simulink model "ACS"  (R2023b)
settings: Solver=FixedStepDiscrete  StartTime=0.0  StopTime=10000  FixedStep=0.01  MaxStep=10  RelTol=1e-5  AbsTol=1e-5  EnableMultiTasking=on
InitFcn:
  | initialization
undefined symbols (not defined in the file): A, AE, air_density, altitude, c_diffus, c_spec, CD, Cell_Area, CM_mm01, CM_mm02, CM_mm03, CO_mm01, CO_mm02, CO_mm03, cos50, cosines, dip_coel, dip_long, DiscIntNeverNeededParam, E_EOL, H0, inc, Inertia_tensor, K_l, k_pb, k_pe, kelly, light_speed, m_m, M_SR, magnitude, MM_Working, MT_Working, N_B, Ncell_Xn, Ncell_Xp, Ncell_Yn, Ncell_Yp, Ncell_Zn, Ncell_Zp, NX, NY, NZ, omega_BI_B0, omega_e, omega_o, omega_tx, omega_ty, omega_tz, quat_0, r, r_cm_B, r_cp_a_B, r_cp_s_B, RAAN_rt, Re, t0, TA_0, theta_g0
libraries: simulink x20, vrlib x5
(part 2 of 3)

== system ACS/Satellite/Magnetorquers/Magnetorquers4 ==
  MT : Inport
  Abs1 : Abs  SaturateOnIntegerOverflow=off
  Constant1 : Constant  Value=0
  Constant4 : Constant  Value=0.0511597
  Constant5 : Constant  Value=24.7613/15/22
  Discrete-Time Integrator1 : DiscreteIntegrator  InitialConditionSource=external  SampleTime=-1  ICPrevOutput=DiscIntNeverNeededParam  ICPrevScaledInput=DiscIntNeverNeededParam
  Gain5 : Gain  Gain=1/15
  Gain6 : Gain  Gain=0.06
  Gain7 : Gain  Gain=22
  Product : Product  Inputs=*/
  Product1 : Product  Inputs=*/
  Sum : Sum  Inputs=+-
  MM_Am2 : Outport  VectorParamsAs1DForOutWhenUnconnected=off
  MM_W : Outport  Port=2  VectorParamsAs1DForOutWhenUnconnected=off
  wires:
  MT/1 -> Product/1
  Constant4/1 -> Product1/2
  Constant1/1 -> Discrete-Time Integrator1/2
  Discrete-Time Integrator1/1 -> MM_Am2/1, Abs1/1, Product1/1
  Product/1 -> Sum/1
  Sum/1 -> Discrete-Time Integrator1/1
  Product1/1 -> Sum/2
  Constant5/1 -> Product/2
  Abs1/1 -> Gain5/1
  Gain5/1 -> Gain6/1
  Gain6/1 -> Gain7/1
  Gain7/1 -> MM_W/1

== system ACS/Satellite/OBC/Data Adquisition ==
  PP_W : Inport
  PD_V : Inport  Port=2
  B_b_V : Inport  Port=3
  Bus Creator : BusCreator  Inputs=3
  Bus Selector : BusSelector  OutputSignals=B_MM1,B_MM2,B_MM3
  Constant : Constant  Value=-960.9  OutDataTypeStr=single
  Constant1 : Constant  Value=-960.9  OutDataTypeStr=single
  Constant2 : Constant  Value=1975.166667  OutDataTypeStr=single
  Gain1 : Gain  Gain=363.6733333
  Gain3 : Gain  Gain=1147.5
  Gain4 : Gain  Gain=1147.5
  Saturation : Saturate  UpperLimit=4.4  LowerLimit=1  ZeroCross=off
  Saturation1 : Saturate  UpperLimit=4.4  LowerLimit=1  ZeroCross=off
  Saturation2 : Saturate  UpperLimit=5.6  LowerLimit=-5.4  ZeroCross=off
  Sum : Sum
  Sum1 : Sum
  Sum2 : Sum
  PP_UPC : Outport  VectorParamsAs1DForOutWhenUnconnected=off
  PD_UPC : Outport  Port=2  VectorParamsAs1DForOutWhenUnconnected=off
  B_b_UPC : Outport  Port=3  VectorParamsAs1DForOutWhenUnconnected=off
  wires:
  B_b_V/1 -> Bus Selector/1
  Bus Creator/1 -> B_b_UPC/1
  PD_V/1 -> PD_UPC/1
  PP_W/1 -> PP_UPC/1
  Bus Selector/1 -> Saturation/1  "<B_MM1>"
  Bus Selector/2 -> Saturation1/1  "<B_MM2>"
  Bus Selector/3 -> Saturation2/1  "<B_MM3>"
  Saturation/1 -> Gain3/1
  Sum/1 -> Bus Creator/1
  Saturation1/1 -> Gain4/1
  Saturation2/1 -> Gain1/1
  Sum2/1 -> Bus Creator/3
  Sum1/1 -> Bus Creator/2
  Gain3/1 -> Sum/1
  Gain4/1 -> Sum1/1
  Gain1/1 -> Sum2/1
  Constant/1 -> Sum/2
  Constant1/1 -> Sum1/2
  Constant2/1 -> Sum2/2

== system ACS/Satellite/OBC/Experimentall Attitude Control ==
  PP_UPC : Inport
  PD_UPC : Inport  Port=2
  B_b_UPC : Inport  Port=3
  Constant1 : Constant  Value=0  OutDataTypeStr=single
  Constant3 : Constant  Value=0  OutDataTypeStr=single
  Terminator1 : Terminator
  Terminator2 : Terminator
  Terminator3 : Terminator
  MT : Outport  VectorParamsAs1DForOutWhenUnconnected=off
  RW : Outport  Port=2  VectorParamsAs1DForOutWhenUnconnected=off
  wires:
  B_b_UPC/1 -> Terminator3/1
  PD_UPC/1 -> Terminator1/1
  PP_UPC/1 -> Terminator2/1
  Constant3/1 -> MT/1
  Constant1/1 -> RW/1

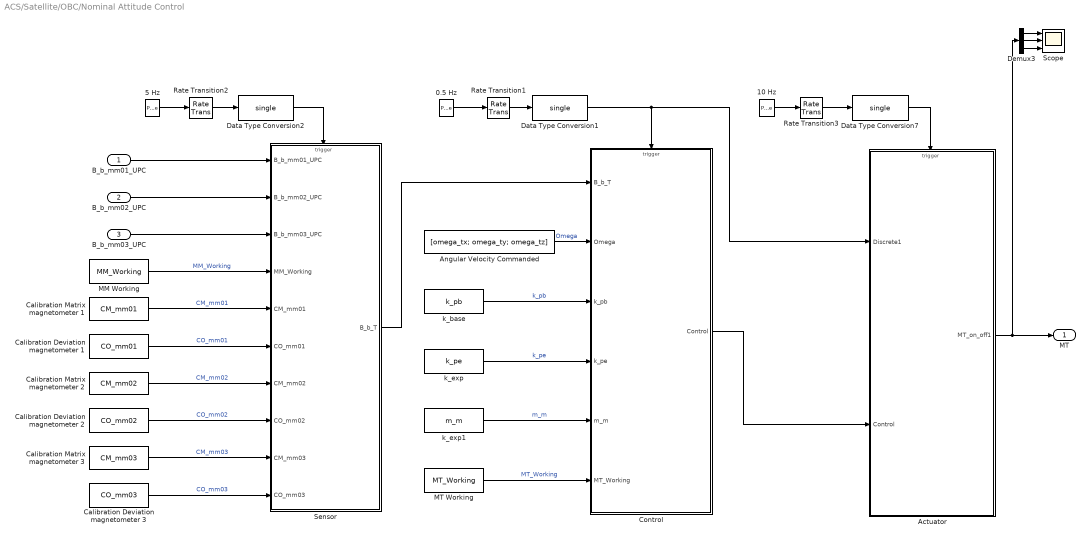
== system ACS/Satellite/OBC/Nominal Attitude Control ==
  B_b_mm01_UPC : Inport
  B_b_mm02_UPC : Inport  Port=2
  B_b_mm03_UPC : Inport  Port=3
  " 5 Hz" : DiscretePulseGenerator  PulseType=Time based  Period=0.2  PulseWidth=50
  0.5 Hz : DiscretePulseGenerator  PulseType=Time based  PulseWidth=25  PhaseDelay=1
  10 Hz : DiscretePulseGenerator  PulseType=Time based  Period=0.2  PulseWidth=50
  Actuator : Subsystem
  Angular Velocity Commanded : Constant  Value=[omega_tx; omega_ty; omega_tz]  OutDataTypeStr=single
  Calibration Deviation magnetometer 1 : Constant  Value=CO_mm01  OutDataTypeStr=single
  Calibration Deviation magnetometer 2 : Constant  Value=CO_mm02  OutDataTypeStr=single
  Calibration Deviation magnetometer 3 : Constant  Value=CO_mm03  OutDataTypeStr=single
  Calibration Matrix magnetometer 1 : Constant  Value=CM_mm01  OutDataTypeStr=single
  Calibration Matrix magnetometer 2 : Constant  Value=CM_mm02  OutDataTypeStr=single
  Calibration Matrix magnetometer 3 : Constant  Value=CM_mm03  OutDataTypeStr=single
  Control : Subsystem
  Data Type Conversion1 : DataTypeConversion  OutDataTypeStr=single  SampleTime=0.1  SaturateOnIntegerOverflow=off  RndMeth=Floor
  Data Type Conversion2 : DataTypeConversion  OutDataTypeStr=single  SampleTime=0.1  SaturateOnIntegerOverflow=off  RndMeth=Floor
  Data Type Conversion7 : DataTypeConversion  OutDataTypeStr=single  SampleTime=0.1  SaturateOnIntegerOverflow=off  RndMeth=Floor
  Demux3 : Demux  Outputs=3
  MM Working : Constant  Value=MM_Working  OutDataTypeStr=single
  MT Working : Constant  Value=MT_Working  OutDataTypeStr=single
  Rate Transition1 : RateTransition  OutPortSampleTime=0.1
  Rate Transition2 : RateTransition  OutPortSampleTime=0.1
  Rate Transition3 : RateTransition  OutPortSampleTime=0.1
  Scope : Scope  NumInputPorts=3
  Sensor : Subsystem
  k_base : Constant  Value=k_pb  OutDataTypeStr=single
  k_exp : Constant  Value=k_pe  OutDataTypeStr=single
  k_exp1 : Constant  Value=m_m  OutDataTypeStr=single
  MT : Outport  VectorParamsAs1DForOutWhenUnconnected=off
  wires:
  Control/1(Control) -> Actuator/2(Control)
  0.5 Hz/1 -> Rate Transition1/1
  10 Hz/1 -> Rate Transition3/1
  Sensor/1(B_b_T) -> Control/1(B_b_T)
  B_b_mm01_UPC/1 -> Sensor/1(B_b_mm01_UPC)
  Data Type Conversion7/1 -> Actuator/Trigger
  Data Type Conversion1/1 -> Control/Trigger, Actuator/1(Discrete1)
  " 5 Hz"/1 -> Rate Transition2/1
  Data Type Conversion2/1 -> Sensor/Trigger
  MM Working/1 -> Sensor/4(MM_Working)  "MM_Working"
  Calibration Matrix magnetometer 1/1 -> Sensor/5(CM_mm01)  "CM_mm01"
  Calibration Deviation magnetometer 1/1 -> Sensor/6(CO_mm01)  "CO_mm01"
  Calibration Matrix magnetometer 2/1 -> Sensor/7(CM_mm02)  "CM_mm02"
  Calibration Deviation magnetometer 2/1 -> Sensor/8(CO_mm02)  "CO_mm02"
  Calibration Matrix magnetometer 3/1 -> Sensor/9(CM_mm03)  "CM_mm03"
  Calibration Deviation magnetometer 3/1 -> Sensor/10(CO_mm03)  "CO_mm03"
  Angular Velocity Commanded/1 -> Control/2(Omega)  "Omega"
  k_base/1 -> Control/3(k_pb)  "k_pb"
  k_exp/1 -> Control/4(k_pe)  "k_pe"
  k_exp1/1 -> Control/5(m_m)  "m_m"
  MT Working/1 -> Control/6(MT_Working)  "MT_Working"
  B_b_mm02_UPC/1 -> Sensor/2(B_b_mm02_UPC)
  B_b_mm03_UPC/1 -> Sensor/3(B_b_mm03_UPC)
  Rate Transition2/1 -> Data Type Conversion2/1
  Rate Transition1/1 -> Data Type Conversion1/1
  Rate Transition3/1 -> Data Type Conversion7/1
  Actuator/1(MT_on_off1) -> MT/1, Demux3/1
  Demux3/3 -> Scope/3
  Demux3/2 -> Scope/2
  Demux3/1 -> Scope/1

== system ACS/Satellite/Photodiodes/Measurements ==
  V : Inport
  Trigger : TriggerPort  VariantControl=(inherit)
  V_V : Outport  VectorParamsAs1DForOutWhenUnconnected=off
  wires:
  V/1 -> V_V/1

== system ACS/Satellite/Photodiodes/Sun ==
  Sol_b_W : Inport
  Add : Sum  Inputs=+++
  Add1 : Sum  Inputs=2
  Compare To Zero : simulink/Logic and Bit Operations/Compare To Zero  relop===  OutDataTypeStr=uint8  ZeroCross=off
  Demux : Demux  Outputs=3
  Math Function : Math  Operator=magnitude^2  SignedPower=on
  Math Function1 : Math  Operator=magnitude^2  SignedPower=on
  Math Function2 : Math  Operator=magnitude^2  SignedPower=on
  Math Function3 : Math  Operator=sqrt  SignedPower=on
  Product4 : Product  Inputs=*/  RndMeth=Zero
  Solar_Direction_b : Outport  VectorParamsAs1DForOutWhenUnconnected=off
  Solar_Flux_W : Outport  Port=2  VectorParamsAs1DForOutWhenUnconnected=off
  wires:
  Demux/1 -> Math Function/1
  Demux/2 -> Math Function1/1
  Math Function/1 -> Add/1
  Math Function1/1 -> Add/2
  Add/1 -> Math Function3/1
  Math Function3/1 -> Add1/1, Solar_Flux_W/1, Compare To Zero/1
  Demux/3 -> Math Function2/1
  Math Function2/1 -> Add/3
  Sol_b_W/1 -> Product4/1, Demux/1
  Product4/1 -> Solar_Direction_b/1
  Add1/1 -> Product4/2
  Compare To Zero/1 -> Add1/2

== system ACS/Satellite/Photodiodes/Voltage ==
  note: fi: angle between earth-sun vector and
      | normal vector of the solar array
  Earth-Sun B : Inport
  Solar Constant : Inport  Port=2
  eclipse : Inport  Port=3
  Constant1 : Constant  Value=NZ
  Constant2 : Constant  Value=NY
  Constant3 : Constant  Value=NX
  Dot Product1 : DotProduct  OutDataTypeStr=Inherit: Inherit via internal rule
  Dot Product2 : DotProduct  OutDataTypeStr=Inherit: Inherit via internal rule
  Dot Product3 : DotProduct  OutDataTypeStr=Inherit: Inherit via internal rule
  Power Generated : Subsystem
  Product3 : Product  Inputs=**  RndMeth=Zero
  factor of view X : Subsystem
  factor of view Y : Subsystem
  factor of view Z : Subsystem
  norm : Subsystem
  norm1 : Subsystem
  norm2 : Subsystem
  norm3 : Subsystem
  norm4 : Subsystem
  norm5 : Subsystem
  PD_V : Outport  VectorParamsAs1DForOutWhenUnconnected=off
  wires:
  norm3/1(2) -> Dot Product2/2
  norm2/1(2) -> Dot Product2/1
  norm1/1(2) -> Dot Product1/2
  norm/1(2) -> Dot Product1/1
  factor of view Z/1(FV) -> Power Generated/3(Cos fi NZ)
  factor of view Y/1(FV) -> Power Generated/2(Cos fi NY)
  Dot Product2/1 -> factor of view Z/1(cos (fi))  "cos fi"
  Dot Product1/1 -> factor of view Y/1(cos (fi))  "cos fi"
  Constant1/1 -> norm2/1(1)
  Constant2/1 -> norm/1(1)
  norm5/1(2) -> Dot Product3/2
  norm4/1(2) -> Dot Product3/1
  Dot Product3/1 -> factor of view X/1(cos (fi))  "cos fi"
  Constant3/1 -> norm4/1(1)
  Earth-Sun B/1 -> norm5/1(1), norm1/1(1), norm3/1(1)
  factor of view X/1(FV) -> Power Generated/1(Cos fi NX)
  Power Generated/1(Voltage) -> Product3/1
  Solar Constant/1 -> Power Generated/4(Solar_constant)
  Product3/1 -> PD_V/1
  eclipse/1 -> Product3/2

== system ACS/Satellite/Solar_Panels/Measurements ==
  V : Inport
  Trigger : TriggerPort  TriggerType=falling  VariantControl=(inherit)
  V_V : Outport  VectorParamsAs1DForOutWhenUnconnected=off
  wires:
  V/1 -> V_V/1

== system ACS/Satellite/Solar_Panels/Power ==
  note: fi: angle between earth-sun vector and
      | normal vector of the solar array
  Earth-Sun B : Inport
  Solar Constant : Inport  Port=2
  eclipse : Inport  Port=3
  Constant1 : Constant  Value=NZ
  Constant2 : Constant  Value=NY
  Constant3 : Constant  Value=NX
  Dot Product1 : DotProduct  OutDataTypeStr=Inherit: Inherit via internal rule
  Dot Product2 : DotProduct  OutDataTypeStr=Inherit: Inherit via internal rule
  Dot Product3 : DotProduct  OutDataTypeStr=Inherit: Inherit via internal rule
  Power Generated : Subsystem
  Product2 : Product  Inputs=**  RndMeth=Zero
  factor of view X : Subsystem
  factor of view Y : Subsystem
  factor of view Z : Subsystem
  norm : Subsystem
  norm1 : Subsystem
  norm2 : Subsystem
  norm3 : Subsystem
  norm4 : Subsystem
  norm5 : Subsystem
  Power_each_W : Outport  VectorParamsAs1DForOutWhenUnconnected=off
  wires:
  factor of view X/1(FV) -> Power Generated/1(Cos fi NX)
  Earth-Sun B/1 -> norm3/1(1), norm1/1(1), norm5/1(1)
  Constant3/1 -> norm4/1(1)
  Dot Product3/1 -> factor of view X/1(cos (fi))  "cos fi"
  norm4/1(2) -> Dot Product3/1
  norm5/1(2) -> Dot Product3/2
  Constant2/1 -> norm/1(1)
  Constant1/1 -> norm2/1(1)
  Dot Product1/1 -> factor of view Y/1(cos (fi))  "cos fi"
  Dot Product2/1 -> factor of view Z/1(cos (fi))  "cos fi"
  factor of view Y/1(FV) -> Power Generated/2(Cos fi NY)
  factor of view Z/1(FV) -> Power Generated/3(Cos fi NZ)
  norm/1(2) -> Dot Product1/1
  norm1/1(2) -> Dot Product1/2
  norm2/1(2) -> Dot Product2/1
  norm3/1(2) -> Dot Product2/2
  Solar Constant/1 -> Power Generated/4(Solar Constant)
  eclipse/1 -> Product2/2
  Product2/1 -> Power_each_W/1
  Power Generated/1(Power_each_W) -> Product2/1

== system ACS/Satellite/Solar_Panels/Power Generated ==
  Sol_b_W : Inport
  Add : Sum  Inputs=+++
  Add1 : Sum  Inputs=2
  Compare To Zero : simulink/Logic and Bit Operations/Compare To Zero  relop===  OutDataTypeStr=uint8  ZeroCross=off
  Demux : Demux  Outputs=3
  Math Function : Math  Operator=magnitude^2  SignedPower=on
  Math Function1 : Math  Operator=magnitude^2  SignedPower=on
  Math Function2 : Math  Operator=magnitude^2  SignedPower=on
  Math Function3 : Math  Operator=sqrt  SignedPower=on
  Product4 : Product  Inputs=*/  RndMeth=Zero
  Solar_Direction_b : Outport  VectorParamsAs1DForOutWhenUnconnected=off
  Solar_Flux_W : Outport  Port=2  VectorParamsAs1DForOutWhenUnconnected=off
  wires:
  Demux/1 -> Math Function/1
  Demux/2 -> Math Function1/1
  Math Function/1 -> Add/1
  Math Function1/1 -> Add/2
  Add/1 -> Math Function3/1
  Math Function3/1 -> Add1/1, Solar_Flux_W/1, Compare To Zero/1
  Demux/3 -> Math Function2/1
  Math Function2/1 -> Add/3
  Sol_b_W/1 -> Product4/1, Demux/1
  Product4/1 -> Solar_Direction_b/1
  Add1/1 -> Product4/2
  Compare To Zero/1 -> Add1/2

== system ACS/Sun1/Solar Rays Direction/Eclipse_ ==
  Earth-Sun B : Inport
  C_BV : Inport  Port=2
  Compare to : simulink/Logic and Bit Operations/Compare To Constant  relop=>  const=cos(AE)  OutDataTypeStr=uint8  ZeroCross=off
  Dot Product1 : DotProduct  OutDataTypeStr=Inherit: Inherit via internal rule
  Product1 : Product  Multiplication=Matrix(*)  RndMeth=Zero
  norm : Subsystem
  norm1 : Subsystem
  sat_earth vector in local vertical reference system : Constant  Value=[0 ;0 ;1]  VectorParams1D=off
  eclipse : Outport  VectorParamsAs1DForOutWhenUnconnected=off
  wires:
  Product1/1 -> norm1/1(1)
  norm/1(2) -> Dot Product1/1  "sat-sun"
  Earth-Sun B/1 -> norm/1(1)
  norm1/1(2) -> Dot Product1/2  "sat-earth"
  Compare to/1 -> eclipse/1
  Dot Product1/1 -> Compare to/1  "cos alpha"
  sat_earth vector in local vertical reference system/1 -> Product1/2
  C_BV/1 -> Product1/1

== system ACS/Sun1/Solar Rays Direction/Solar direction in inertial ==
  delta : Inport
  epsilon : Inport  Port=2
  gamma : Inport  Port=3
  Divide : Product  Inputs=**  Multiplication=Matrix(*)
  Inertial 2 Orbital Plane1 : Subsystem  mask(Inertial 2 Mean Sun){}
      mask help:
      | This Block performs the transformation matrix using angle between vernal equinox and Earth-MeanSun (gamma) for transformation from Inertial coordinate frame to Mean Sun coordinate frame.
      | The origin of  Mean Sun coordinate frame is on Earth center and its x-axis is toward Mean Sun and its z-axis is toward Earth North Pole.
      | Where Mean Sun is a virtual Sun which is rotating around Earth in a circular orbit with 1 year period.
      |
      |             [  c(gamma)        S(gamma)     0 ]
      | C_MSI =[ -S(gamma)      C(gamma)      0 ]
      |              [  0                        0                 1 ]
      mask Display:
      | port_label('input', 1, '\gamma','texmode','on')
      | port_label('output', 1, 'C_I^{MS}','texmode','on')
      | disp('Inertial 2 Mean Sun')
  Math Function : Math  Operator=transpose  SignedPower=on
  Mux : Mux  Inputs=3
  Product1 : Product  RndMeth=Zero
  Product2 : Product  RndMeth=Zero
  Trigonometric Function : Trigonometry  Operator=cos
  Trigonometric Function1 : Trigonometry  Operator=cos
  Trigonometric Function2 : Trigonometry  Operator=cos
  Trigonometric Function3 : Trigonometry
  Trigonometric Function4 : Trigonometry
  S_ES_I : Outport  VectorParamsAs1DForOutWhenUnconnected=off
  wires:
  Math Function/1 -> Divide/1
  gamma/1 -> Inertial 2 Orbital Plane1/1(gamma)
  Divide/1 -> S_ES_I/1
  Inertial 2 Orbital Plane1/1(C_MSI) -> Math Function/1
  Mux/1 -> Divide/2
  Trigonometric Function4/1 -> Mux/3
  Product1/1 -> Mux/2
  Product2/1 -> Mux/1
  Trigonometric Function1/1 -> Product2/2
  Trigonometric Function/1 -> Product2/1
  epsilon/1 -> Trigonometric Function1/1, Trigonometric Function3/1
  delta/1 -> Trigonometric Function4/1, Trigonometric Function/1, Trigonometric Function2/1
  Trigonometric Function2/1 -> Product1/1
  Trigonometric Function3/1 -> Product1/2

== system ACS/Sun1/Sun Annalema/Calculating Sun position ==
  Time_passed from J2000.0 : Inport
  Declination (Deg) : Subsystem
  Ecliptic Longitude (Deg) : Subsystem
  Ecuation of Time (Deg) : Subsystem
  Mean anomaly of the Sun (Deg) : Subsystem
  Mean longitude of the Sun (Deg) : Subsystem
  Obliquity of ecliptic (Deg) : Subsystem
  Right ascension (Deg) : Subsystem
  gamma_deg : Outport  VectorParamsAs1DForOutWhenUnconnected=off
  EOT_deg : Outport  Port=2  VectorParamsAs1DForOutWhenUnconnected=off
  declination_deg : Outport  Port=3  VectorParamsAs1DForOutWhenUnconnected=off
  wires:
  Time_passed from J2000.0/1 -> Mean longitude of the Sun (Deg)/1(n), Mean anomaly of the Sun (Deg)/1(n), Obliquity of ecliptic (Deg)/1(n)  "n of days from J2000.0"
  Mean longitude of the Sun (Deg)/1(L) -> Ecliptic Longitude (Deg)/1(L), Ecuation of Time (Deg)/1(L), gamma_deg/1
  Ecliptic Longitude (Deg)/1(Lambda) -> Declination (Deg)/1(Lambda), Right ascension (Deg)/1(Lambda)
  Mean anomaly of the Sun (Deg)/1(g) -> Ecliptic Longitude (Deg)/2(g)
  Obliquity of ecliptic (Deg)/1(epsilon) -> Right ascension (Deg)/2(epsion), Declination (Deg)/2(epsilon)
  Right ascension (Deg)/1(alpha) -> Ecuation of Time (Deg)/2(alpha)
  Ecuation of Time (Deg)/1(E) -> EOT_deg/1
  Declination (Deg)/1(delta) -> declination_deg/1

== system ACS/Earth/Simple model of Earth's Magnetic Field1/Simple model of Earth's Magnetic Field1/Inertial 2 Orbital Plane1 ==
  long_lat : Inport
  Constant4 : Constant  Value=0
  Fcn : Fcn  Expr=-cos(u(1))*sin(u(2))
  Fcn1 : Fcn  Expr=-sin(u(1))
  Fcn2 : Fcn  Expr=-cos(u(1))*cos(u(2))
  Fcn3 : Fcn  Expr=-sin(u(1))*sin(u(2))
  Fcn4 : Fcn  Expr=cos(u(1))
  Fcn5 : Fcn  Expr=-sin(u(1))*cos(u(2))
  Fcn6 : Fcn  Expr=cos(u(2))
  Fcn7 : Fcn  Expr=-sin(u(2))
  Mux : Mux  Inputs=9
  Reshape : Reshape  OutputDimensionality=Customize  OutputDimensions=[3,3]
  C_NED_ECEF : Outport  VectorParamsAs1DForOutWhenUnconnected=off
  wires:
  Mux/1 -> Reshape/1
  Fcn/1 -> Mux/1
  long_lat/1 -> Fcn/1, Fcn1/1, Fcn2/1, Fcn3/1, Fcn4/1, Fcn5/1, Fcn6/1, Fcn7/1
  Fcn1/1 -> Mux/2
  Fcn2/1 -> Mux/3
  Fcn3/1 -> Mux/4
  Fcn4/1 -> Mux/5
  Fcn5/1 -> Mux/6
  Fcn7/1 -> Mux/9
  Reshape/1 -> C_NED_ECEF/1
  Fcn6/1 -> Mux/7
  Constant4/1 -> Mux/8

== system ACS/Earth/Simple model of Earth's Magnetic Field1/Simple model of Earth's Magnetic Field1/Simple Magnetc Field ==
  dd_ECEF : Inport
  C_NED_ECEF : Inport  Port=2
  Enable : EnablePort
  " 3nd gaussian coefficient2" : Constant  Value=H0
  " 3nd gaussian coefficient3" : Constant  Value=Re
  " 3nd gaussian coefficient4" : Constant  Value=3
  " R_NED" : Constant  Value=[0;0;-r]
  Divide1 : Product  Inputs=**
  Divide16 : Product  Inputs=**  Multiplication=Matrix(*)
  Divide2 : Product  Inputs=**  Multiplication=Matrix(*)
  Earths magnetic field in Inertial frame1 : Subsystem
  Gain : Gain  Gain=1e-9
  Math Function1 : Math  Operator=transpose  SignedPower=on
  Math Function5 : Math  Operator=pow  SignedPower=on
  B_NED : Outport  VectorParamsAs1DForOutWhenUnconnected=off
  B_ECEF : Outport  Port=2  VectorParamsAs1DForOutWhenUnconnected=off
  wires:
  " 3nd gaussian coefficient2"/1 -> Gain/1
  Divide1/1 -> Earths magnetic field in Inertial frame1/3(TS)
  Math Function5/1 -> Divide1/1
  " 3nd gaussian coefficient4"/1 -> Math Function5/2
  " 3nd gaussian coefficient3"/1 -> Math Function5/1
  " R_NED"/1 -> Divide16/2
  Math Function1/1 -> Divide16/1
  Gain/1 -> Divide1/2
  C_NED_ECEF/1 -> Math Function1/1, Divide2/1
  dd_ECEF/1 -> Earths magnetic field in Inertial frame1/2(dd_ECEF)
  Earths magnetic field in Inertial frame1/1(B_ECEF) -> B_ECEF/1, Divide2/2
  Divide16/1 -> Earths magnetic field in Inertial frame1/1(R_ECEF)
  Divide2/1 -> B_NED/1

== system ACS/Earth/Simple model of Earth's Magnetic Field1/Simple model of Earth's Magnetic Field1/dipole direction in geocentric inertial frame ==
  theta_md : Inport
  phi_md : Inport  Port=2
  Fcn : Fcn  Expr=sin(u(1))*cos(u(2))
  Fcn1 : Fcn  Expr=sin(u(1))*sin(u(2))
  Fcn2 : Fcn  Expr=cos(u(1))
  Mux : Mux  Inputs=3
  Mux1 : Mux  Inputs=2
  Dipol_direction_ECEF : Outport  VectorParamsAs1DForOutWhenUnconnected=off
  wires:
  Fcn2/1 -> Mux/3
  Fcn1/1 -> Mux/2
  Fcn/1 -> Mux/1
  Mux1/1 -> Fcn2/1, Fcn1/1, Fcn/1
  phi_md/1 -> Mux1/2
  theta_md/1 -> Mux1/1
  Mux/1 -> Dipol_direction_ECEF/1

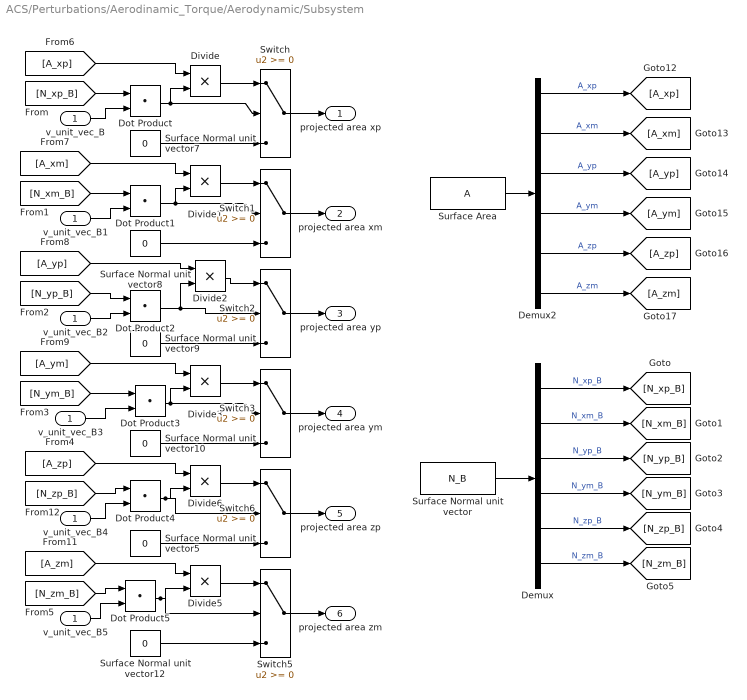
== system ACS/Perturbations/Aerodinamic_Torque/Aerodynamic/Subsystem ==
  v_unit_vec_B : Inport
  Demux : Demux  Outputs=6
  Demux2 : Demux  Outputs=6
  Divide{,1..3,5..6} (6 alike) : Product  Inputs=**
  Dot Product{,1..5} (6 alike) : DotProduct  OutDataTypeStr=Inherit: Inherit via internal rule
  Surface Area : Constant  Value=A
  Surface Normal unit vector : Constant  Value=N_B
  Surface Normal unit vector{5,7..10,12} (6 alike) : Constant  Value=0
  Switch{,1..3,5..6} (6 alike) : Switch  SaturateOnIntegerOverflow=off  InputSameDT=off
  v_unit_vec_B{1..5} (5 alike) : InportShadow
  projected area xp : Outport  VectorParamsAs1DForOutWhenUnconnected=off
  projected area xm : Outport  Port=2  VectorParamsAs1DForOutWhenUnconnected=off
  projected area yp : Outport  Port=3  VectorParamsAs1DForOutWhenUnconnected=off
  projected area ym : Outport  Port=4  VectorParamsAs1DForOutWhenUnconnected=off
  projected area zp : Outport  Port=5  VectorParamsAs1DForOutWhenUnconnected=off
  projected area zm : Outport  Port=6  VectorParamsAs1DForOutWhenUnconnected=off
  wires:
  Surface Normal unit vector7/1 -> Switch/3
  [A_xp] -> Divide/1
  Divide/1 -> Switch/1
  Surface Normal unit vector8/1 -> Switch1/3
  [A_xm] -> Divide1/1
  Divide1/1 -> Switch1/1
  Surface Normal unit vector9/1 -> Switch2/3
  [A_yp] -> Divide2/1
  Divide2/1 -> Switch2/1
  Surface Normal unit vector10/1 -> Switch3/3
  [A_ym] -> Divide3/1
  Divide3/1 -> Switch3/1
  Surface Normal unit vector12/1 -> Switch5/3
  [A_zm] -> Divide5/1
  Divide5/1 -> Switch5/1
  Surface Normal unit vector5/1 -> Switch6/3
  [A_zp] -> Divide6/1
  Divide6/1 -> Switch6/1
  Switch/1 -> projected area xp/1
  Switch1/1 -> projected area xm/1
  Switch2/1 -> projected area yp/1
  Switch3/1 -> projected area ym/1
  Switch6/1 -> projected area zp/1
  Switch5/1 -> projected area zm/1
  Demux/1 -> [N_xp_B]  "N_xp_B"
  Demux/2 -> [N_xm_B]  "N_xm_B"
  Demux/3 -> [N_yp_B]  "N_yp_B"
  Demux/4 -> [N_ym_B]  "N_ym_B"
  Demux/5 -> [N_zp_B]  "N_zp_B"
  Demux/6 -> [N_zm_B]  "N_zm_B"
  Surface Area/1 -> Demux2/1
  Demux2/1 -> [A_xp]  "A_xp"
  Demux2/2 -> [A_xm]  "A_xm"
  Demux2/3 -> [A_yp]  "A_yp"
  Demux2/4 -> [A_ym]  "A_ym"
  Demux2/5 -> [A_zp]  "A_zp"
  Demux2/6 -> [A_zm]  "A_zm"
  Surface Normal unit vector/1 -> Demux/1
  [N_xp_B] -> Dot Product/1
  v_unit_vec_B/1 -> Dot Product/2
  Dot Product/1 -> Divide/2, Switch/2
  [N_xm_B] -> Dot Product1/1
  v_unit_vec_B1/1 -> Dot Product1/2
  Dot Product1/1 -> Divide1/2, Switch1/2
  [N_yp_B] -> Dot Product2/1
  v_unit_vec_B2/1 -> Dot Product2/2
  Dot Product2/1 -> Switch2/2, Divide2/2
  [N_ym_B] -> Dot Product3/1
  v_unit_vec_B3/1 -> Dot Product3/2
  Dot Product3/1 -> Divide3/2, Switch3/2
  [N_zp_B] -> Dot Product4/1
  v_unit_vec_B4/1 -> Dot Product4/2
  Dot Product4/1 -> Divide6/2, Switch6/2
  [N_zm_B] -> Dot Product5/1
  v_unit_vec_B5/1 -> Dot Product5/2
  Dot Product5/1 -> Divide5/2, Switch5/2

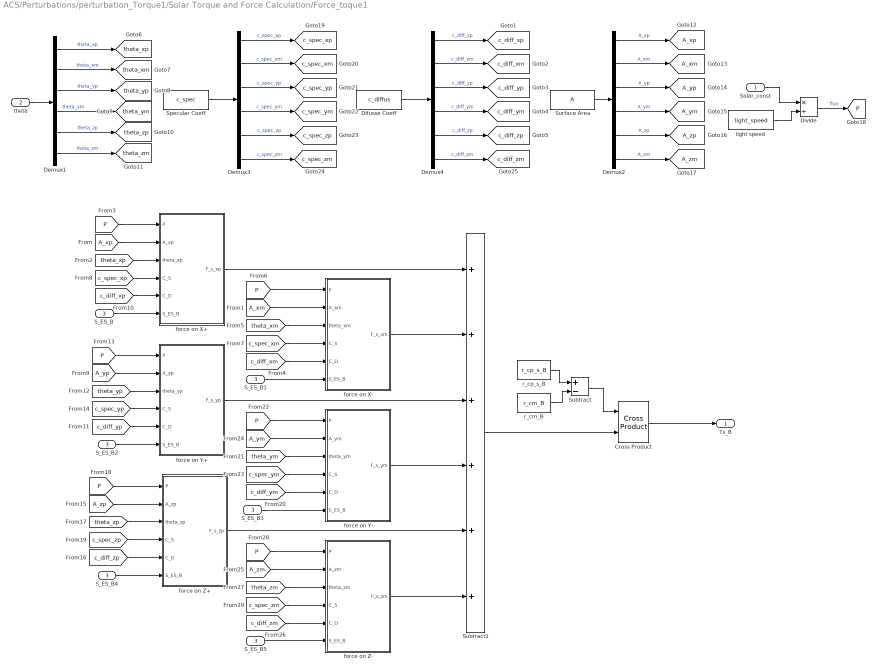
== system ACS/Perturbations/perturbation_Torque1/Solar Torque and Force Calculation/Force_toque1 ==
  Solar_const : Inport
  theta : Inport  Port=2
  S_ES_B : Inport  Port=3
  Cross Product : vrlib/Utilities/Cross Product
  Demux{1..4} (4 alike) : Demux  Outputs=6
  Difusse Coeff : Constant  Value=c_diffus
  Divide : Product  Inputs=*/
  S_ES_B{1..5} (5 alike) : InportShadow  Port=3
  Specular Coeff : Constant  Value=c_spec
  Subtract : Sum  Inputs=+-
  Subtract1 : Sum  Inputs=++++++
  Surface Area : Constant  Value=A
  force on X+ : Subsystem
  force on X- : Subsystem
  force on Y+ : Subsystem
  force on Y- : Subsystem
  force on Z+ : Subsystem
  force on Z- : Subsystem
  light speed : Constant  Value=light_speed
  r_cm_B : Constant  Value=r_cm_B
  r_cp_s_B : Constant  Value=r_cp_s_B
  Ts_B : Outport  VectorParamsAs1DForOutWhenUnconnected=off
  tag scope: A_xm=global, A_xp=global, A_ym=global, A_yp=global, A_zm=global, A_zp=global, P=global, c_diff_xm=global, c_diff_xp=global, c_diff_ym=global, c_diff_yp=global, c_diff_zm=global, c_diff_zp=global, c_spec_xm=global, c_spec_xp=global, c_spec_ym=global, c_spec_yp=global, c_spec_zm=global, c_spec_zp=global, theta_xm=global, theta_xp=global, theta_ym=global, theta_yp=global, theta_zm=global, theta_zp=global
  wires:
  [c_diff_ym] -> force on Y-/5(C_D)
  [c_spec_ym] -> force on Y-/4(C_S)
  [theta_ym] -> force on Y-/3(theta_ym)
  [A_ym] -> force on Y-/2(A_ym)
  [P] -> force on Y-/1(P)
  [c_diff_zm] -> force on Z-/5(C_D)
  [c_spec_zm] -> force on Z-/4(C_S)
  [theta_zm] -> force on Z-/3(theta_zm)
  [A_zm] -> force on Z-/2(A_zm)
  [P] -> force on Z-/1(P)
  [c_diff_zp] -> force on Z+/5(C_D)
  [c_spec_zp] -> force on Z+/4(C_S)
  [theta_zp] -> force on Z+/3(theta_zp)
  [A_zp] -> force on Z+/2(A_zp)
  [P] -> force on Z+/1(P)
  [c_diff_yp] -> force on Y+/5(C_D)
  [c_spec_yp] -> force on Y+/4(C_S)
  [theta_yp] -> force on Y+/3(theta_yp)
  [A_yp] -> force on Y+/2(A_yp)
  [P] -> force on Y+/1(P)
  [c_diff_xm] -> force on X-/5(C_D)
  [c_spec_xm] -> force on X-/4(C_S)
  [theta_xm] -> force on X-/3(theta_xm)
  [A_xm] -> force on X-/2(A_xm)
  [P] -> force on X-/1(P)
  S_ES_B5/1 -> force on Z-/6(S_ES_B)
  S_ES_B1/1 -> force on X-/6(S_ES_B)
  S_ES_B3/1 -> force on Y-/6(S_ES_B)
  S_ES_B4/1 -> force on Z+/6(S_ES_B)
  S_ES_B2/1 -> force on Y+/6(S_ES_B)
  [c_diff_xp] -> force on X+/5(C_D)
  Demux4/1 -> [c_diff_xp]  "c_diff_xp"
  Demux4/2 -> [c_diff_xm]  "c_diff_xm"
  Demux4/3 -> [c_diff_yp]  "c_diff_yp"
  Demux4/4 -> [c_diff_ym]  "c_diff_ym"
  Demux4/5 -> [c_diff_zp]  "c_diff_zp"
  Demux4/6 -> [c_diff_zm]  "c_diff_zm"
  Difusse Coeff/1 -> Demux4/1
  r_cp_s_B/1 -> Subtract/1
  r_cm_B/1 -> Subtract/2
  [P] -> force on X+/1(P)
  [A_xp] -> force on X+/2(A_xp)
  S_ES_B/1 -> force on X+/6(S_ES_B)
  force on X+/1(F_s_xp) -> Subtract1/1
  force on Y+/1(F_s_yp) -> Subtract1/3
  force on Z+/1(F_s_zp) -> Subtract1/5
  force on X-/1(F_s_xm) -> Subtract1/2
  force on Y-/1(F_s_ym) -> Subtract1/4
  force on Z-/1(F_s_zm) -> Subtract1/6
  Subtract1/1 -> Cross Product/2
  Subtract/1 -> Cross Product/1
  Cross Product/1 -> Ts_B/1
  [theta_xp] -> force on X+/3(theta_xp)
  [c_spec_xp] -> force on X+/4(C_S)
  Solar_const/1 -> Divide/1
  light speed/1 -> Divide/2
  theta/1 -> Demux1/1
  Surface Area/1 -> Demux2/1
  Demux2/1 -> [A_xp]  "A_xp"
  Demux2/2 -> [A_xm]  "A_xm"
  Demux2/3 -> [A_yp]  "A_yp"
  Demux2/4 -> [A_ym]  "A_ym"
  Demux2/5 -> [A_zp]  "A_zp"
  Demux2/6 -> [A_zm]  "A_zm"
  Demux1/1 -> [theta_xp]  "theta_xp"
  Demux1/2 -> [theta_xm]  "theta_xm"
  Demux1/3 -> [theta_yp]  "theta_yp"
  Demux1/4 -> [theta_ym]  "theta_ym"
  Demux1/5 -> [theta_zp]  "theta_zp"
  Demux1/6 -> [theta_zm]  "theta_zm"
  Divide/1 -> [P]  "flux"
  Demux3/1 -> [c_spec_xp]  "c_spec_xp"
  Demux3/2 -> [c_spec_xm]  "c_spec_xm"
  Demux3/3 -> [c_spec_yp]  "c_spec_yp"
  Demux3/4 -> [c_spec_ym]  "c_spec_ym"
  Demux3/5 -> [c_spec_zp]  "c_spec_zp"
  Demux3/6 -> [c_spec_zm]  "c_spec_zm"
  Specular Coeff/1 -> Demux3/1

== system ACS/Perturbations/perturbation_Torque1/Solar Torque and Force Calculation/Surface-Sun Angle ==
  S_ES_B : Inport
  Dot Product{,1..5} (6 alike) : DotProduct  OutDataTypeStr=Inherit: Inherit via internal rule
  Mux : Mux  Inputs=6
  Selector : Selector  InputPortWidth=18  IndexOptions=Index vector (dialog)  Indices=[1 2 3]  OutputSizes=1
  Selector1 : Selector  InputPortWidth=18  IndexOptions=Index vector (dialog)  Indices=[4 5 6]  OutputSizes=1
  Selector2 : Selector  InputPortWidth=18  IndexOptions=Index vector (dialog)  Indices=[7 8 9]  OutputSizes=1
  Selector3 : Selector  InputPortWidth=18  IndexOptions=Index vector (dialog)  Indices=[10 11 12]  OutputSizes=1
  Selector4 : Selector  InputPortWidth=18  IndexOptions=Index vector (dialog)  Indices=[13 14 15]  OutputSizes=1
  Selector5 : Selector  InputPortWidth=18  IndexOptions=Index vector (dialog)  Indices=[16 17 18]  OutputSizes=1
  Surface Normal unit vector : Constant  Value=N_B
  Trigonometric Function{,1..5} (6 alike) : Trigonometry  Operator=acos
  theta : Outport  VectorParamsAs1DForOutWhenUnconnected=off
  wires:
  Selector5/1 -> Dot Product5/2  "N_zm_B"
  Selector4/1 -> Dot Product4/2  "N_zp_B"
  Selector3/1 -> Dot Product3/2  "N_ym_B"
  Selector2/1 -> Dot Product2/2  "N_yp_B"
  Selector1/1 -> Dot Product1/2  "N_xm_B"
  Selector/1 -> Dot Product/2  "N_xp_B"
  S_ES_B/1 -> Dot Product5/1, Dot Product4/1, Dot Product3/1, Dot Product2/1, Dot Product1/1, Dot Product/1
  Dot Product5/1 -> Trigonometric Function5/1
  Dot Product4/1 -> Trigonometric Function4/1
  Dot Product3/1 -> Trigonometric Function3/1
  Dot Product2/1 -> Trigonometric Function2/1
  Dot Product1/1 -> Trigonometric Function1/1
  Dot Product/1 -> Trigonometric Function/1
  Mux/1 -> theta/1
  Trigonometric Function/1 -> Mux/1
  Trigonometric Function1/1 -> Mux/2
  Trigonometric Function2/1 -> Mux/3
  Trigonometric Function3/1 -> Mux/4
  Trigonometric Function4/1 -> Mux/5
  Trigonometric Function5/1 -> Mux/6
  Surface Normal unit vector/1 -> Selector3/1, Selector4/1, Selector5/1, Selector2/1, Selector1/1, Selector/1

== system ACS/Satellite/OBC/Nominal Attitude Control/Actuator ==
  Discrete1 : Inport
  Control : Inport  Port=2
  Trigger : TriggerPort  TriggerType=either  VariantControl=(inherit)
  Abs1 : Abs  SaturateOnIntegerOverflow=off
  Compare To Zero : simulink/Logic and Bit Operations/Compare To Zero  relop=>=  OutDataTypeStr=uint8  ZeroCross=off
  Constant1 : Constant  OutDataTypeStr=single
  Discrete-Time Integrator : DiscreteIntegrator  ExternalReset=rising  InitialCondition=0.1  SampleTime=-1  ICPrevOutput=DiscIntNeverNeededParam  ICPrevScaledInput=DiscIntNeverNeededParam
  Product : Product  RndMeth=Zero
  Product1 : Product  RndMeth=Zero
  Sign : Signum
  Sum : Sum  Inputs=+-
  MT_on_off1 : Outport  VectorParamsAs1DForOutWhenUnconnected=off
  wires:
  Discrete-Time Integrator/1 -> Sum/2
  Product1/1 -> Abs1/1, Sign/1
  Sum/1 -> Compare To Zero/1
  Compare To Zero/1 -> Product/2
  Product/1 -> MT_on_off1/1
  Sign/1 -> Product/1
  Discrete1/1 -> Product1/1
  Abs1/1 -> Discrete-Time Integrator/2, Sum/1
  Control/1 -> Product1/2
  Constant1/1 -> Discrete-Time Integrator/1

== system ACS/Satellite/OBC/Nominal Attitude Control/Control ==
  B_b_T : Inport
  Omega : Inport  Port=2
  k_pb : Inport  Port=3
  k_pe : Inport  Port=4
  m_m : Inport  Port=5
  MT_Working : Inport  Port=6
  Trigger : TriggerPort  VariantControl=(inherit)
  Control law : Subsystem
  If Fail Recalculate : Subsystem
  Limitation : Subsystem
  Magnetic field calculation : Subsystem
  discretization : Subsystem
  Control : Outport  VectorParamsAs1DForOutWhenUnconnected=off
  wires:
  Magnetic field calculation/2(B_med) -> If Fail Recalculate/2(B_b_T), Control law/2(B)
  Magnetic field calculation/1(B_dot) -> Control law/1(B_dot)
  B_b_T/1 -> Magnetic field calculation/1(B_b_T1)
  MT_Working/1 -> If Fail Recalculate/3(Working)
  Limitation/1(MT) -> discretization/1(PD)
  Control law/1(M) -> If Fail Recalculate/1(M)
  If Fail Recalculate/1(I_A) -> Limitation/1(M)
  discretization/1(MT) -> Control/1
  Omega/1 -> Control law/3(omega)
  m_m/1 -> discretization/2(m_m), Limitation/2("m_m ")
  k_pb/1 -> Control law/4(k_pb)
  k_pe/1 -> Control law/5(k_pe)

== system ACS/Satellite/OBC/Nominal Attitude Control/Sensor ==
  B_b_mm01_UPC : Inport
  B_b_mm02_UPC : Inport  Port=2
  B_b_mm03_UPC : Inport  Port=3
  MM_Working : Inport  Port=4
  CM_mm01 : Inport  Port=5
  CO_mm01 : Inport  Port=6
  CM_mm02 : Inport  Port=7
  CO_mm02 : Inport  Port=8
  CM_mm03 : Inport  Port=9
  CO_mm03 : Inport  Port=10
  Trigger : TriggerPort  VariantControl=(inherit)
  Average : Subsystem
  "Magnetometer data conversion " : Subsystem
  Memory : Subsystem
  B_b_T : Outport  VectorParamsAs1DForOutWhenUnconnected=off
  wires:
  B_b_mm01_UPC/1 -> "Magnetometer data conversion "/1(B_b_mm01_UPC)
  Memory/1(B_b_T_1s) -> B_b_T/1
  Average/1(B_b_T_1s) -> Memory/1(B_b_T)
  "Magnetometer data conversion "/1(B_b_T) -> Average/1(B_b_T)
  MM_Working/1 -> Average/2(MM_working)
  CM_mm01/1 -> "Magnetometer data conversion "/4(CM_mm01)
  CO_mm01/1 -> "Magnetometer data conversion "/5(CO_mm01)
  CM_mm02/1 -> "Magnetometer data conversion "/6(CM_mm02)
  CO_mm02/1 -> "Magnetometer data conversion "/7(CO_mm02)
  CM_mm03/1 -> "Magnetometer data conversion "/8(CM_mm03)
  CO_mm03/1 -> "Magnetometer data conversion "/9(CO_mm03)
  B_b_mm02_UPC/1 -> "Magnetometer data conversion "/2(B_b_mm02_UPC)
  B_b_mm03_UPC/1 -> "Magnetometer data conversion "/3(B_b_mm03_UPC)

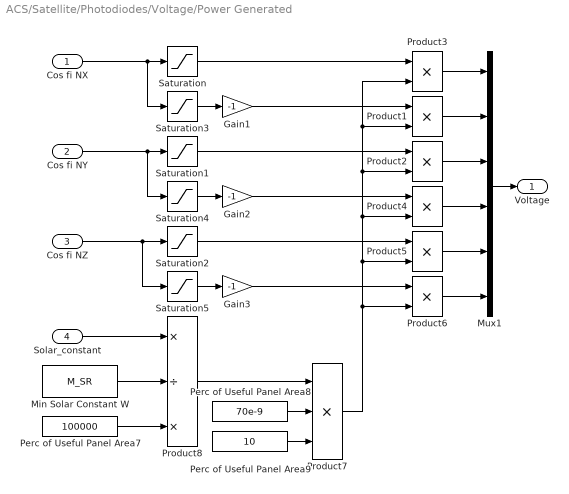
== system ACS/Satellite/Photodiodes/Voltage/Power Generated ==
  Cos fi NX : Inport
  Cos fi NY : Inport  Port=2
  Cos fi NZ : Inport  Port=3
  Solar_constant : Inport  Port=4
  Gain1 : Gain  Gain=-1
  Gain2 : Gain  Gain=-1
  Gain3 : Gain  Gain=-1
  Min Solar Constant W : Constant  Value=M_SR
  Mux1 : Mux  Inputs=6
  Perc of Useful Panel Area7 : Constant  Value=100000
  Perc of Useful Panel Area8 : Constant  Value=70e-9
  Perc of Useful Panel Area9 : Constant  Value=10
  Product{1..6} (6 alike) : Product  RndMeth=Zero
  Product7 : Product  Inputs=3  RndMeth=Zero
  Product8 : Product  Inputs=*/*  RndMeth=Zero
  Saturation : Saturate  UpperLimit=1  LowerLimit=0
  Saturation1 : Saturate  UpperLimit=1  LowerLimit=0
  Saturation2 : Saturate  UpperLimit=1  LowerLimit=0
  Saturation3 : Saturate  UpperLimit=0  LowerLimit=-1
  Saturation4 : Saturate  UpperLimit=0  LowerLimit=-1
  Saturation5 : Saturate  UpperLimit=0  LowerLimit=-1
  Voltage : Outport  VectorParamsAs1DForOutWhenUnconnected=off
  wires:
  Cos fi NX/1 -> Saturation/1, Saturation3/1
  Product3/1 -> Mux1/1
  Cos fi NY/1 -> Saturation1/1, Saturation4/1
  Cos fi NZ/1 -> Saturation2/1, Saturation5/1
  Product1/1 -> Mux1/2
  Product2/1 -> Mux1/3
  Product4/1 -> Mux1/4
  Product5/1 -> Mux1/5
  Product6/1 -> Mux1/6
  Saturation/1 -> Product3/1
  Saturation1/1 -> Product2/1
  Saturation2/1 -> Product5/1
  Saturation3/1 -> Gain1/1
  Saturation4/1 -> Gain2/1
  Saturation5/1 -> Gain3/1
  Gain1/1 -> Product1/1
  Gain2/1 -> Product4/1
  Gain3/1 -> Product6/1
  Mux1/1 -> Voltage/1
  Perc of Useful Panel Area7/1 -> Product8/3
  Perc of Useful Panel Area8/1 -> Product7/2
  Perc of Useful Panel Area9/1 -> Product7/3
  Product7/1 -> Product6/2, Product5/2, Product4/2, Product2/2, Product1/2, Product3/2
  Solar_constant/1 -> Product8/1
  Product8/1 -> Product7/1
  Min Solar Constant W/1 -> Product8/2

== system ACS/Satellite/Photodiodes/Voltage/factor of view X ==
  cos (fi) : Inport
  Abs1 : Abs  SaturateOnIntegerOverflow=off
  Compare to cos (55) : simulink/Logic and Bit Operations/Compare To Constant  relop=>=  const=cos(55*pi/180)  OutDataTypeStr=uint8  ZeroCross=off
  Product : Product  RndMeth=Zero
  FV : Outport  VectorParamsAs1DForOutWhenUnconnected=off
  wires:
  Compare to cos (55)/1 -> Product/2
  cos (fi)/1 -> Abs1/1, Product/1
  Abs1/1 -> Compare to cos (55)/1
  Product/1 -> FV/1

== system ACS/Satellite/Photodiodes/Voltage/factor of view Y ==
  cos (fi) : Inport
  Abs1 : Abs  SaturateOnIntegerOverflow=off
  Compare to cos (55) : simulink/Logic and Bit Operations/Compare To Constant  relop=>=  const=cos(55*pi/180)  OutDataTypeStr=uint8  ZeroCross=off
  Product : Product  RndMeth=Zero
  FV : Outport  VectorParamsAs1DForOutWhenUnconnected=off
  wires:
  Product/1 -> FV/1
  Abs1/1 -> Compare to cos (55)/1
  cos (fi)/1 -> Product/1, Abs1/1
  Compare to cos (55)/1 -> Product/2

== system ACS/Satellite/Photodiodes/Voltage/factor of view Z ==
  cos (fi) : Inport
  Abs1 : Abs  SaturateOnIntegerOverflow=off
  Compare to cos (55) : simulink/Logic and Bit Operations/Compare To Constant  relop=>=  const=cos(55*pi/180)  OutDataTypeStr=uint8  ZeroCross=off
  Product : Product  RndMeth=Zero
  FV : Outport  VectorParamsAs1DForOutWhenUnconnected=off
  wires:
  Compare to cos (55)/1 -> Product/2
  cos (fi)/1 -> Abs1/1, Product/1
  Abs1/1 -> Compare to cos (55)/1
  Product/1 -> FV/1

== system ACS/Satellite/Photodiodes/Voltage/norm ==
  1 : Inport
  Add1 : Sum  Inputs=+
  Math Function2 : Math  Operator=square  SignedPower=on
  Math Function3 : Math  Operator=sqrt  SignedPower=on
  Product1 : Product  Inputs=*/  RndMeth=Zero
  2 : Outport  VectorParamsAs1DForOutWhenUnconnected=off
  wires:
  Product1/1 -> 2/1
  Math Function2/1 -> Add1/1
  Add1/1 -> Math Function3/1
  Math Function3/1 -> Product1/2
  1/1 -> Product1/1, Math Function2/1

== system ACS/Satellite/Photodiodes/Voltage/norm1 ==
  1 : Inport
  Add1 : Sum  Inputs=+
  Math Function2 : Math  Operator=square  SignedPower=on
  Math Function3 : Math  Operator=sqrt  SignedPower=on
  Product1 : Product  Inputs=*/  RndMeth=Zero
  2 : Outport  VectorParamsAs1DForOutWhenUnconnected=off
  wires:
  1/1 -> Math Function2/1, Product1/1
  Math Function3/1 -> Product1/2
  Add1/1 -> Math Function3/1
  Math Function2/1 -> Add1/1
  Product1/1 -> 2/1

== system ACS/Satellite/Photodiodes/Voltage/norm2 ==
  1 : Inport
  Add1 : Sum  Inputs=+
  Math Function2 : Math  Operator=square  SignedPower=on
  Math Function3 : Math  Operator=sqrt  SignedPower=on
  Product1 : Product  Inputs=*/  RndMeth=Zero
  2 : Outport  VectorParamsAs1DForOutWhenUnconnected=off
  wires:
  1/1 -> Math Function2/1, Product1/1
  Math Function3/1 -> Product1/2
  Add1/1 -> Math Function3/1
  Math Function2/1 -> Add1/1
  Product1/1 -> 2/1

== system ACS/Satellite/Photodiodes/Voltage/norm3 ==
  1 : Inport
  Add1 : Sum  Inputs=+
  Math Function2 : Math  Operator=square  SignedPower=on
  Math Function3 : Math  Operator=sqrt  SignedPower=on
  Product1 : Product  Inputs=*/  RndMeth=Zero
  2 : Outport  VectorParamsAs1DForOutWhenUnconnected=off
  wires:
  Product1/1 -> 2/1
  Math Function2/1 -> Add1/1
  Add1/1 -> Math Function3/1
  Math Function3/1 -> Product1/2
  1/1 -> Product1/1, Math Function2/1

== system ACS/Satellite/Photodiodes/Voltage/norm4 ==
  1 : Inport
  Add1 : Sum  Inputs=+
  Math Function2 : Math  Operator=square  SignedPower=on
  Math Function3 : Math  Operator=sqrt  SignedPower=on
  Product1 : Product  Inputs=*/  RndMeth=Zero
  2 : Outport  VectorParamsAs1DForOutWhenUnconnected=off
  wires:
  1/1 -> Math Function2/1, Product1/1
  Math Function3/1 -> Product1/2
  Add1/1 -> Math Function3/1
  Math Function2/1 -> Add1/1
  Product1/1 -> 2/1

== system ACS/Satellite/Photodiodes/Voltage/norm5 ==
  1 : Inport
  Add1 : Sum  Inputs=+
  Math Function2 : Math  Operator=square  SignedPower=on
  Math Function3 : Math  Operator=sqrt  SignedPower=on
  Product1 : Product  Inputs=*/  RndMeth=Zero
  2 : Outport  VectorParamsAs1DForOutWhenUnconnected=off
  wires:
  Product1/1 -> 2/1
  Math Function2/1 -> Add1/1
  Add1/1 -> Math Function3/1
  Math Function3/1 -> Product1/2
  1/1 -> Product1/1, Math Function2/1

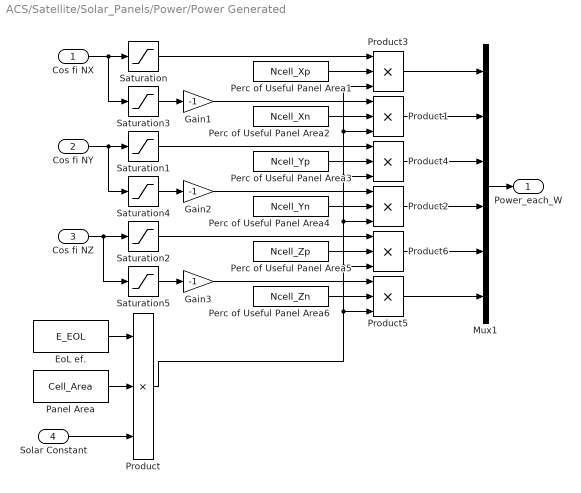
== system ACS/Satellite/Solar_Panels/Power/Power Generated ==
  Cos fi NX : Inport
  Cos fi NY : Inport  Port=2
  Cos fi NZ : Inport  Port=3
  Solar Constant : Inport  Port=4
  EoL ef. : Constant  Value=E_EOL
  Gain1 : Gain  Gain=-1
  Gain2 : Gain  Gain=-1
  Gain3 : Gain  Gain=-1
  Mux1 : Mux  Inputs=6
  Panel Area : Constant  Value=Cell_Area
  Perc of Useful Panel Area1 : Constant  Value=Ncell_Xp
  Perc of Useful Panel Area2 : Constant  Value=Ncell_Xn
  Perc of Useful Panel Area3 : Constant  Value=Ncell_Yp
  Perc of Useful Panel Area4 : Constant  Value=Ncell_Yn
  Perc of Useful Panel Area5 : Constant  Value=Ncell_Zp
  Perc of Useful Panel Area6 : Constant  Value=Ncell_Zn
  Product{,1..6} (7 alike) : Product  Inputs=3  RndMeth=Zero
  Saturation : Saturate  UpperLimit=1  LowerLimit=0
  Saturation1 : Saturate  UpperLimit=1  LowerLimit=0
  Saturation2 : Saturate  UpperLimit=1  LowerLimit=0
  Saturation3 : Saturate  UpperLimit=0  LowerLimit=-1
  Saturation4 : Saturate  UpperLimit=0  LowerLimit=-1
  Saturation5 : Saturate  UpperLimit=0  LowerLimit=-1
  Power_each_W : Outport  VectorParamsAs1DForOutWhenUnconnected=off
  wires:
  Mux1/1 -> Power_each_W/1
  Gain3/1 -> Product5/1
  Gain2/1 -> Product2/1
  Gain1/1 -> Product1/1
  Saturation5/1 -> Gain3/1
  Saturation4/1 -> Gain2/1
  Saturation3/1 -> Gain1/1
  Saturation2/1 -> Product6/1
  Saturation1/1 -> Product4/1
  Saturation/1 -> Product3/1
  Product/1 -> Product5/3, Product6/3, Product2/3, Product4/3, Product1/3, Product3/3
  Perc of Useful Panel Area6/1 -> Product5/2
  Perc of Useful Panel Area5/1 -> Product6/2
  Cos fi NZ/1 -> Saturation5/1, Saturation2/1
  Perc of Useful Panel Area4/1 -> Product2/2
  Perc of Useful Panel Area3/1 -> Product4/2
  Cos fi NY/1 -> Saturation4/1, Saturation1/1
  Perc of Useful Panel Area2/1 -> Product1/2
  Perc of Useful Panel Area1/1 -> Product3/2
  Cos fi NX/1 -> Saturation3/1, Saturation/1
  EoL ef./1 -> Product/1
  Panel Area/1 -> Product/2
  Solar Constant/1 -> Product/3
  Product5/1 -> Mux1/6
  Product6/1 -> Mux1/5
  Product2/1 -> Mux1/4
  Product4/1 -> Mux1/3
  Product1/1 -> Mux1/2
  Product3/1 -> Mux1/1

== system ACS/Satellite/Solar_Panels/Power/factor of view X ==
  cos (fi) : Inport
  Abs1 : Abs  SaturateOnIntegerOverflow=off
  Compare to cos (50) : simulink/Logic and Bit Operations/Compare To Constant  relop=>=  const=cos50  OutDataTypeStr=uint8  ZeroCross=off
  Kelly Cosine1 : Lookup  InputValues=cosines  Table=kelly  SaturateOnIntegerOverflow=off
  Logical Operator : Logic  Operator=NOT  AllPortsSameDT=off  OutDataTypeStr=boolean
  Product : Product  RndMeth=Zero
  Product1 : Product  RndMeth=Zero
  Product2 : Product  RndMeth=Zero
  Saturation : Saturate  UpperLimit=1  LowerLimit=0
  Sign : Signum
  Sum : Sum
  FV : Outport  VectorParamsAs1DForOutWhenUnconnected=off
  wires:
  Sign/1 -> Product2/1
  Product2/1 -> FV/1
  Abs1/1 -> Compare to cos (50)/1, Kelly Cosine1/1, Product/1
  Saturation/1 -> Product1/2
  Kelly Cosine1/1 -> Saturation/1
  Product1/1 -> Sum/2
  Product/1 -> Sum/1
  Logical Operator/1 -> Product1/1
  Sum/1 -> Product2/2
  cos (fi)/1 -> Sign/1, Abs1/1
  Compare to cos (50)/1 -> Logical Operator/1, Product/2

== system ACS/Satellite/Solar_Panels/Power/factor of view Y ==
  cos (fi) : Inport
  Abs1 : Abs  SaturateOnIntegerOverflow=off
  Compare to cos (50) : simulink/Logic and Bit Operations/Compare To Constant  relop=>=  const=cos50  OutDataTypeStr=uint8  ZeroCross=off
  Kelly Cosine1 : Lookup  InputValues=cosines  Table=kelly  SaturateOnIntegerOverflow=off
  Logical Operator : Logic  Operator=NOT  AllPortsSameDT=off  OutDataTypeStr=boolean
  Product : Product  RndMeth=Zero
  Product1 : Product  RndMeth=Zero
  Product2 : Product  RndMeth=Zero
  Saturation : Saturate  UpperLimit=1  LowerLimit=0
  Sign : Signum
  Sum : Sum
  FV : Outport  VectorParamsAs1DForOutWhenUnconnected=off
  wires:
  Compare to cos (50)/1 -> Product/2, Logical Operator/1
  cos (fi)/1 -> Abs1/1, Sign/1
  Sum/1 -> Product2/2
  Logical Operator/1 -> Product1/1
  Product/1 -> Sum/1
  Product1/1 -> Sum/2
  Kelly Cosine1/1 -> Saturation/1
  Saturation/1 -> Product1/2
  Abs1/1 -> Product/1, Kelly Cosine1/1, Compare to cos (50)/1
  Product2/1 -> FV/1
  Sign/1 -> Product2/1

== system ACS/Satellite/Solar_Panels/Power/factor of view Z ==
  cos (fi) : Inport
  Abs1 : Abs  SaturateOnIntegerOverflow=off
  Compare to cos (50) : simulink/Logic and Bit Operations/Compare To Constant  relop=>=  const=cos50  OutDataTypeStr=uint8  ZeroCross=off
  Kelly Cosine1 : Lookup  InputValues=cosines  Table=kelly  SaturateOnIntegerOverflow=off
  Logical Operator : Logic  Operator=NOT  AllPortsSameDT=off  OutDataTypeStr=boolean
  Product : Product  RndMeth=Zero
  Product1 : Product  RndMeth=Zero
  Product2 : Product  RndMeth=Zero
  Saturation : Saturate  UpperLimit=1  LowerLimit=0
  Sign : Signum
  Sum : Sum
  FV : Outport  VectorParamsAs1DForOutWhenUnconnected=off
  wires:
  Sign/1 -> Product2/1
  Product2/1 -> FV/1
  Abs1/1 -> Compare to cos (50)/1, Kelly Cosine1/1, Product/1
  Saturation/1 -> Product1/2
  Kelly Cosine1/1 -> Saturation/1
  Product1/1 -> Sum/2
  Product/1 -> Sum/1
  Logical Operator/1 -> Product1/1
  Sum/1 -> Product2/2
  cos (fi)/1 -> Sign/1, Abs1/1
  Compare to cos (50)/1 -> Logical Operator/1, Product/2

== system ACS/Satellite/Solar_Panels/Power/norm ==
  1 : Inport
  Add1 : Sum  Inputs=+
  Math Function2 : Math  Operator=square  SignedPower=on
  Math Function3 : Math  Operator=sqrt  SignedPower=on
  Product1 : Product  Inputs=*/  RndMeth=Zero
  2 : Outport  VectorParamsAs1DForOutWhenUnconnected=off
  wires:
  1/1 -> Math Function2/1, Product1/1
  Math Function3/1 -> Product1/2
  Add1/1 -> Math Function3/1
  Math Function2/1 -> Add1/1
  Product1/1 -> 2/1

== system ACS/Satellite/Solar_Panels/Power/norm1 ==
  1 : Inport
  Add1 : Sum  Inputs=+
  Math Function2 : Math  Operator=square  SignedPower=on
  Math Function3 : Math  Operator=sqrt  SignedPower=on
  Product1 : Product  Inputs=*/  RndMeth=Zero
  2 : Outport  VectorParamsAs1DForOutWhenUnconnected=off
  wires:
  Product1/1 -> 2/1
  Math Function2/1 -> Add1/1
  Add1/1 -> Math Function3/1
  Math Function3/1 -> Product1/2
  1/1 -> Product1/1, Math Function2/1

== system ACS/Satellite/Solar_Panels/Power/norm2 ==
  1 : Inport
  Add1 : Sum  Inputs=+
  Math Function2 : Math  Operator=square  SignedPower=on
  Math Function3 : Math  Operator=sqrt  SignedPower=on
  Product1 : Product  Inputs=*/  RndMeth=Zero
  2 : Outport  VectorParamsAs1DForOutWhenUnconnected=off
  wires:
  Product1/1 -> 2/1
  Math Function2/1 -> Add1/1
  Add1/1 -> Math Function3/1
  Math Function3/1 -> Product1/2
  1/1 -> Product1/1, Math Function2/1

== system ACS/Satellite/Solar_Panels/Power/norm3 ==
  1 : Inport
  Add1 : Sum  Inputs=+
  Math Function2 : Math  Operator=square  SignedPower=on
  Math Function3 : Math  Operator=sqrt  SignedPower=on
  Product1 : Product  Inputs=*/  RndMeth=Zero
  2 : Outport  VectorParamsAs1DForOutWhenUnconnected=off
  wires:
  1/1 -> Math Function2/1, Product1/1
  Math Function3/1 -> Product1/2
  Add1/1 -> Math Function3/1
  Math Function2/1 -> Add1/1
  Product1/1 -> 2/1

== system ACS/Satellite/Solar_Panels/Power/norm4 ==
  1 : Inport
  Add1 : Sum  Inputs=+
  Math Function2 : Math  Operator=square  SignedPower=on
  Math Function3 : Math  Operator=sqrt  SignedPower=on
  Product1 : Product  Inputs=*/  RndMeth=Zero
  2 : Outport  VectorParamsAs1DForOutWhenUnconnected=off
  wires:
  Product1/1 -> 2/1
  Math Function2/1 -> Add1/1
  Add1/1 -> Math Function3/1
  Math Function3/1 -> Product1/2
  1/1 -> Product1/1, Math Function2/1

== system ACS/Satellite/Solar_Panels/Power/norm5 ==
  1 : Inport
  Add1 : Sum  Inputs=+
  Math Function2 : Math  Operator=square  SignedPower=on
  Math Function3 : Math  Operator=sqrt  SignedPower=on
  Product1 : Product  Inputs=*/  RndMeth=Zero
  2 : Outport  VectorParamsAs1DForOutWhenUnconnected=off
  wires:
  1/1 -> Math Function2/1, Product1/1
  Math Function3/1 -> Product1/2
  Add1/1 -> Math Function3/1
  Math Function2/1 -> Add1/1
  Product1/1 -> 2/1

== system ACS/Sun1/Solar Rays Direction/Eclipse_/norm ==
  1 : Inport
  Add1 : Sum  Inputs=+
  Math Function2 : Math  Operator=square  SignedPower=on
  Math Function3 : Math  Operator=sqrt  SignedPower=on
  Product1 : Product  Inputs=*/  RndMeth=Zero
  2 : Outport  VectorParamsAs1DForOutWhenUnconnected=off
  wires:
  Product1/1 -> 2/1
  Math Function2/1 -> Add1/1
  Add1/1 -> Math Function3/1
  Math Function3/1 -> Product1/2
  1/1 -> Product1/1, Math Function2/1

== system ACS/Sun1/Solar Rays Direction/Eclipse_/norm1 ==
  1 : Inport
  Add1 : Sum  Inputs=+
  Math Function2 : Math  Operator=square  SignedPower=on
  Math Function3 : Math  Operator=sqrt  SignedPower=on
  Product1 : Product  Inputs=*/  RndMeth=Zero
  2 : Outport  VectorParamsAs1DForOutWhenUnconnected=off
  wires:
  1/1 -> Math Function2/1, Product1/1
  Math Function3/1 -> Product1/2
  Add1/1 -> Math Function3/1
  Math Function2/1 -> Add1/1
  Product1/1 -> 2/1

== system ACS/Sun1/Solar Rays Direction/Solar direction in inertial/Inertial 2 Orbital Plane1 ==
  gamma : Inport
  Constant1 : Constant  Value=0
  Constant2 : Constant  Value=0
  Constant3 : Constant
  Gain2 : Gain  Gain=-1
  Mux1 : Mux  Inputs=9
  Reshape1 : Reshape  OutputDimensionality=Customize  OutputDimensions=[3,3]
  Trigonometric Function12 : Trigonometry  Operator=cos
  Trigonometric Function13 : Trigonometry
  Trigonometric Function14 : Trigonometry  Operator=cos
  C_MSI : Outport  VectorParamsAs1DForOutWhenUnconnected=off
  wires:
  Mux1/1 -> Reshape1/1
  Trigonometric Function12/1 -> Mux1/1
  Trigonometric Function13/1 -> Gain2/1, Mux1/4
  Gain2/1 -> Mux1/2
  Constant1/1 -> Mux1/3
  Trigonometric Function14/1 -> Mux1/5
  Constant2/1 -> Mux1/6, Mux1/7, Mux1/8
  Constant3/1 -> Mux1/9
  gamma/1 -> Trigonometric Function12/1, Trigonometric Function13/1, Trigonometric Function14/1
  Reshape1/1 -> C_MSI/1

== system ACS/Sun1/Sun Annalema/Calculating Sun position/Declination (Deg) ==
  Lambda : Inport
  epsilon : Inport  Port=2
  Gain1 : Gain  Gain=180/pi
  Gain3 : Gain  Gain=pi/180
  Gain4 : Gain  Gain=pi/180
  Product : Product  RndMeth=Zero
  Trigonometric Function : Trigonometry
  Trigonometric Function1 : Trigonometry
  Trigonometric Function2 : Trigonometry  Operator=asin
  delta : Outport  VectorParamsAs1DForOutWhenUnconnected=off
  wires:
  epsilon/1 -> Gain3/1
  Lambda/1 -> Gain4/1
  Trigonometric Function2/1 -> Gain1/1
  Trigonometric Function/1 -> Product/2
  Trigonometric Function1/1 -> Product/1
  Product/1 -> Trigonometric Function2/1
  Gain1/1 -> delta/1
  Gain3/1 -> Trigonometric Function1/1
  Gain4/1 -> Trigonometric Function/1
